simulink model "ExperimentFourSim"  (R2015a)
settings: Solver=ode45  StartTime=0.0  StopTime=10  RelTol=1e-3
values from neighbouring files (symbols this model uses):
  b = 0.1    [ExperimentFour.m]    (also in ExperimentSix.m = 10; ExperimentTwo.m = 0.9; ExperimentZero.m = a + 2)
  g = 9.8    [ExperimentFour.m]    (also in ExperimentOne.m = ilaplace(G,t))
  I = 0.006    [ExperimentFour.m]
  l = 0.3    [ExperimentFour.m]
  m = 0.2    [ExperimentFour.m]    (also in ExperimentSix.m = 1; ExperimentTwo.m = 2)
  M = 0.5    [ExperimentFour.m]
libraries: dspsrcs4 x1
settings Model: Creator=Abdullah  LastModifiedBy=Abdullah

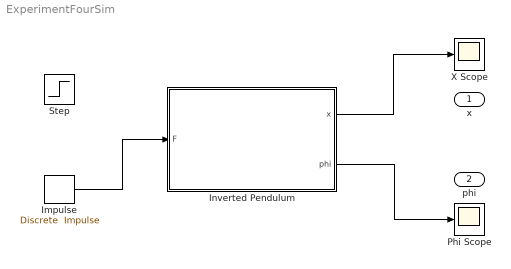
== system ExperimentFourSim ==
  Impulse : dspsrcs4/Discrete  Impulse  Delay=0  SampleTime=1  FrameSample=1  dataType=double  isSigned=on  wordLen=16  udDataType=sfix(16)  fracBitsMode=Best precision  numFracBits=15  OutDataTypeStr=double  LastOutDataTypeStr=double
  Inverted Pendulum : Subsystem
  Phi Scope : Scope
  Step : Step  SampleTime=0
  X Scope : Scope
  x : Outport
  phi : Outport  Port=2
  wires:
  Inverted Pendulum/1(x) -> X Scope/1
  Inverted Pendulum/2(phi) -> Phi Scope/1
  Impulse/1 -> Inverted Pendulum/1(F)

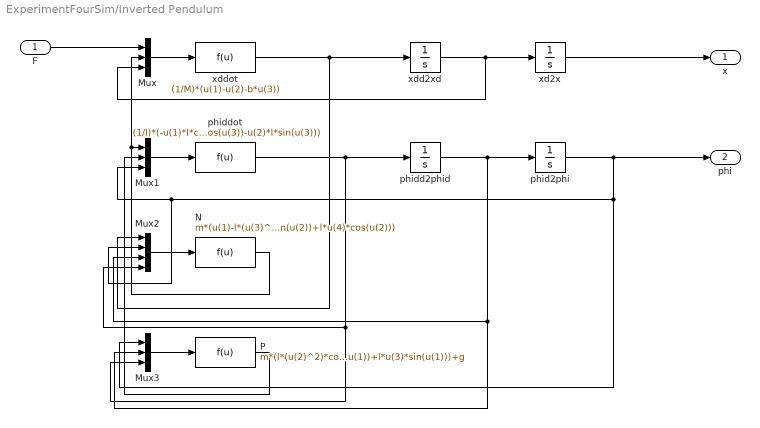
== system ExperimentFourSim/Inverted Pendulum ==
  F : Inport
  Mux : Mux  Inputs=3
  Mux1 : Mux  Inputs=3
  Mux2 : Mux
  Mux3 : Mux  Inputs=3
  N : Fcn  Expr=m*(u(1)-l*(u(3)^2)*sin(u(2))+l*u(4)*cos(u(2)))
  P : Fcn  Expr=m*(l*(u(2)^2)*cos(u(1))+l*u(3)*sin(u(1)))+g
  phid2phi : Integrator
  phidd2phid : Integrator
  phiddot : Fcn  Expr=(1/I)*(-u(1)*l*cos(u(3))-u(2)*l*sin(u(3)))
  xd2x : Integrator
  xdd2xd : Integrator
  xddot : Fcn  Expr=(1/M)*(u(1)-u(2)-b*u(3))
  x : Outport
  phi : Outport  Port=2
  wires:
  xdd2xd/1 -> Mux/3, xd2x/1
  Mux/1 -> xddot/1
  Mux3/1 -> P/1
  P/1 -> Mux1/2
  xddot/1 -> Mux2/1, xdd2xd/1
  phiddot/1 -> Mux3/3, Mux2/4, phidd2phid/1
  xd2x/1 -> x/1
  Mux2/1 -> N/1
  F/1 -> Mux/1
  phid2phi/1 -> phi/1, Mux3/1, Mux2/2, Mux1/3
  N/1 -> Mux1/1, Mux/2
  phidd2phid/1 -> Mux3/2, Mux2/3, phid2phi/1
  Mux1/1 -> phiddot/1
